simulink model "FactorialTask"  (R2021a)
settings: Solver=FixedStepDiscrete  StartTime=0.0  StopTime=10.0  RelTol=1e-3
settings Model: Creator=Dell  LastModifiedBy=Dell
settings OptimizationCC: DefaultParameterBehavior=Inlined  EnhancedBackFolding=on  PassReuseOutputArgsAs=Individual arguments  ZeroExternalMemoryAtStartup=off  ZeroInternalMemoryAtStartup=off  OptimizeBlockOrder=speed  DifferentSizesBufferReuse=on  OptimizationCustomize=off  EfficientTunableParamExpr=on
settings DebuggingCC: ParameterTunabilityLossMsg=error
settings SFSimCC: MATLABDynamicMemAlloc=off
settings RTWCC: SystemTargetFile=ert.tlc  GenCodeOnly=on  TemplateMakefile=ert_default_tmf  GenerateReport=on  IncludeHyperlinkInReport=on  LaunchReport=on  GenerateTraceInfo=on
settings CodeAppCC: ForceParamTrailComments=on  IgnoreCustomStorageClasses=off  OperatorAnnotations=on  SimulinkDataObjDesc=on  SFDataObjDesc=on  InsertBlockDesc=on
settings ERTTargetCC: TargetLangStandard=C99 (ISO)  GenerateSampleERTMain=on  InlinedParameterPlacement=NonHierarchical  ERTCustomFileTemplate=example_file_process.tlc

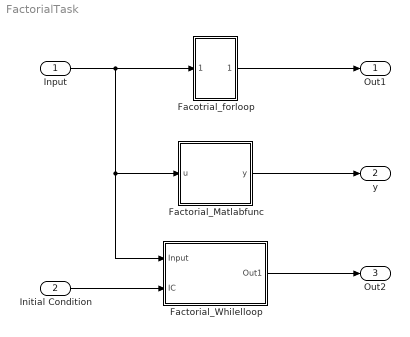
== system FactorialTask ==
  Input : Inport
  Initial Condition : Inport  Port=2
  Facotrial_forloop : Subsystem
  Factorial_Matlabfunc : Subsystem
  Factorial_Whilelloop : Subsystem
  Out1 : Outport
  y : Outport  Port=2
  Out2 : Outport  Port=3
  wires:
  Input/1 -> Factorial_Whilelloop/1(Input), Factorial_Matlabfunc/1(u), Facotrial_forloop/1(In1)
  Facotrial_forloop/1(Out1) -> Out1/1
  Factorial_Matlabfunc/1(y) -> y/1
  Initial Condition/1 -> Factorial_Whilelloop/2(IC)
  Factorial_Whilelloop/1(Out1) -> Out2/1

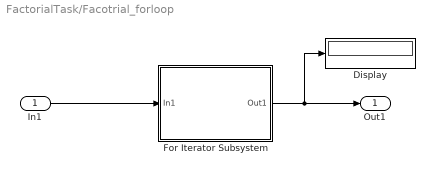
== system FactorialTask/Facotrial_forloop ==
  In1 : Inport
  Display : Display
  For Iterator Subsystem : Subsystem  TreatAsAtomicUnit=on
  Out1 : Outport
  wires:
  For Iterator Subsystem/1(Out1) -> Out1/1, Display/1
  In1/1 -> For Iterator Subsystem/1(In1)

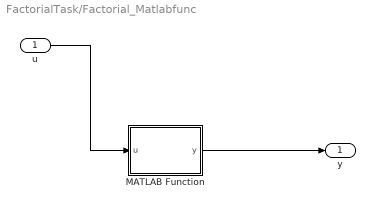
== system FactorialTask/Factorial_Matlabfunc ==
  u : Inport
  MATLAB Function : MATLAB Function  TreatAsAtomicUnit=on
  y : Outport
  wires:
  MATLAB Function/1(y) -> y/1
  u/1 -> MATLAB Function/1(u)

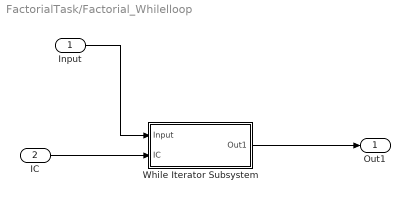
== system FactorialTask/Factorial_Whilelloop ==
  Input : Inport
  IC : Inport  Port=2
  While Iterator Subsystem : Subsystem  TreatAsAtomicUnit=on
  Out1 : Outport
  wires:
  While Iterator Subsystem/1(Out1) -> Out1/1
  IC/1 -> While Iterator Subsystem/2(IC)
  Input/1 -> While Iterator Subsystem/1(Input)

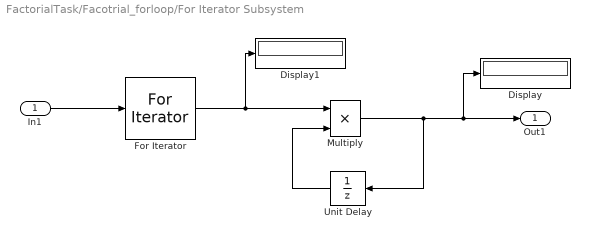
== system FactorialTask/Facotrial_forloop/For Iterator Subsystem ==
  In1 : Inport  OutDataTypeStr=uint8
  Display : Display
  Display1 : Display
  For Iterator : ForIterator  ResetStates=reset  IterationSource=external  IterationVariableDataType=uint8
  Multiply : Product  Inputs=**  OutDataTypeStr=uint8
  Unit Delay : UnitDelay  InitialCondition=1  SampleTime=-1  HasFrameUpgradeWarning=on
  Out1 : Outport  OutDataTypeStr=uint8
  wires:
  For Iterator/1 -> Multiply/1, Display1/1
  Multiply/1 -> Unit Delay/1, Out1/1, Display/1
  Unit Delay/1 -> Multiply/2
  In1/1 -> For Iterator/1

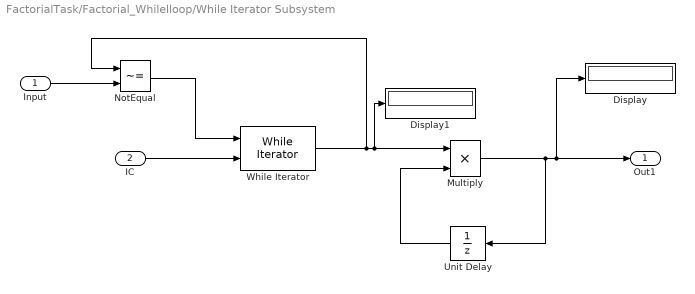
== system FactorialTask/Factorial_Whilelloop/While Iterator Subsystem ==
  Input : Inport
  IC : Inport  Port=2  OutDataTypeStr=boolean
  Display : Display
  Display1 : Display
  Multiply : Product  Inputs=**  OutDataTypeStr=int32
  NotEqual : RelationalOperator  Operator=~=  OutDataTypeStr=boolean  RndMeth=Simplest
  Unit Delay : UnitDelay  InitialCondition=1  SampleTime=-1  HasFrameUpgradeWarning=on
  While Iterator : WhileIterator  MaxIters=-1  ResetStates=reset  ShowIterationPort=on
  Out1 : Outport
  wires:
  IC/1 -> While Iterator/2
  Unit Delay/1 -> Multiply/2
  Multiply/1 -> Unit Delay/1, Display/1, Out1/1
  Input/1 -> NotEqual/2
  NotEqual/1 -> While Iterator/1
  While Iterator/1 -> NotEqual/1, Display1/1, Multiply/1

== matlab function FactorialTask/Factorial_Matlabfunc/MATLAB Function ==
  data: u input; y output
function y = fcn(u)
y=factorial(u);
end
